simulink library "dab"  (Simulink 8.5)
settings: Solver=ode45  SolverMode=SingleTasking  StartTime=0.0  StopTime=10.0  RelTol=1e-3
undefined symbols (not defined in the file or in its folder): den, dx, num
settings Model: Creator=PC  LastModifiedBy=PC

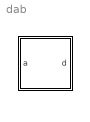
== system dab ==
  "  " : Subsystem  mask(Data Adquisition Board){filter=off, approx=Bessel, order=2, numerator=[], denominator=[], freq=180, resdis=off, vertres=12, xmax=10, winsize=40, G=1.0, fs=60*40}
      mask prompts: filter "Disable Analog Filter"; approx "Filter approximation"; numerator "Free expression filter: numerator(descending order of s)"; denominator "Free expression filter: denominator:"; freq "Cut-off frequency"; resdis "Disable Vertical Resolution"; vertres "Vertical Resolution: No. of bits"; xmax "Vertical Resolution: signal range"; winsize "Window size"; G "Gain"; fs "Sampling frequency"
      mask help: Takes the instantaneous value of the input signal and convert it to the data window of samples.
      mask init:
      | dab1
      mask Help: web(['file:///' which('dab.html')]);
      mask TypeOptions approx: Bessel | Tschebyscheff | Butterworth | free expression
      mask TypeOptions order: 2 | 3 | 4
      mask TypeOptions vertres: 8 | 12 | 16
      mask Display: disp('DAB')

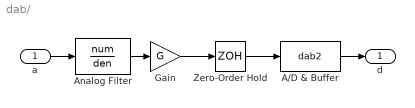
== system dab/   ==
  a : Inport
  A/D & Buffer : S-Function  FunctionName=dab2  Parameters=winsize,fs,dx,resdis
  Analog Filter : TransferFcn  Numerator=num  Denominator=den
  Gain : Gain  Gain=G  SaturateOnIntegerOverflow=on  OutDataTypeStr=Inherit: Same as input  ParamDataTypeStr=Inherit: Same as input
  Zero-Order Hold : ZeroOrderHold  SampleTime=1/fs
  d : Outport  InitialOutput=[zeros(winsize,1)]
  wires:
  Analog Filter/1 -> Gain/1
  Gain/1 -> Zero-Order Hold/1
  Zero-Order Hold/1 -> A/D & Buffer/1
  a/1 -> Analog Filter/1
  A/D & Buffer/1 -> d/1
